simulink model "LT_p2017"  (R2015a)
settings: Solver=ode5  StartTime=0  StopTime=sim_time-1/sr  FixedStep=1/sr  RelTol=1e-3
values from neighbouring files (symbols this model uses):
  par = p.Results.par_fix    [balance_sim.m]
settings Model: Creator=lorenz  LastModifiedBy=lorenz
settings DataIOCC: LimitDataPoints=off  SignalLoggingSaveFormat=ModelDataLogs  SaveOutput=off  SignalLogging=off  DSMLogging=off  SaveTime=off
settings OptimizationCC: OptimizeBlockIOStorage=off  BufferReuse=off  GlobalBufferReuse=off  ExpressionFolding=off  LocalBlockOutputs=off
settings DebuggingCC: UnderspecifiedInitializationDetection=Classic  SolverPrmCheckMsg=warning  InheritedTsInSrcMsg=none  MultiTaskDSMMsg=warning  MultiTaskCondExecSysMsg=none
settings ModelReferenceCC: UpdateModelReferenceTargets=AssumeUpToDate  CheckModelReferenceTargetMessage=warning
settings RTWCC: ProfileTLC=on  RTWUseSimCustomCode=on
settings CodeAppCC: MATLABSourceComments=on

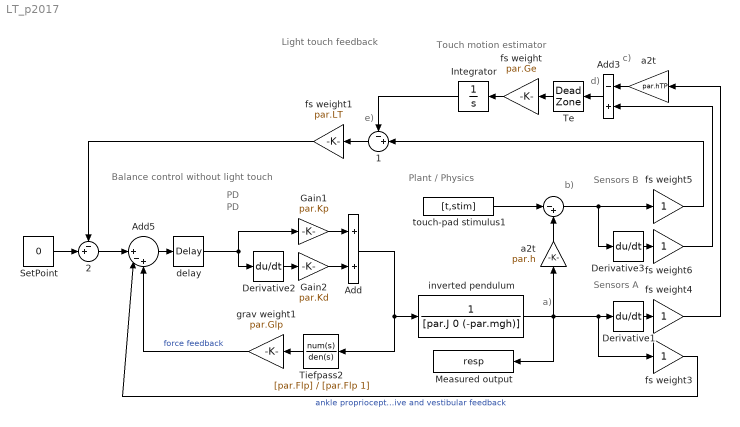
== system LT_p2017 ==
  note: d)
  note: e)
  note: c)
  note: b)
  note: a)
  note: PD
  note: Plant / Physics
  note: Sensors A
  note: Sensors B
  note: Balance control without light touch
  note: PD
  note: Light touch feedback
  note: Touch motion estimator
  " " : Sum  Inputs=|-+
  " 1" : Sum  Inputs=-+|
  " 2" : Sum  Inputs=-+|
  Add : Sum
  Add3 : Sum  Inputs=-+
  Add5 : Sum  Inputs=||+-+
  Derivative1 : Derivative
  Derivative2 : Derivative
  Derivative3 : Derivative
  Gain1 : Gain  Gain=par.Kp
  Gain2 : Gain  Gain=par.Kd
  Integrator : Integrator
  Measured output : ToWorkspace  VariableName=resp  SampleTime=-1
      mask Display: fprintf('measured output')
  SetPoint : Constant  Value=0
  Te : DeadZone  LowerValue=-par.te  UpperValue=par.te  LinearizeAsGain=off
  Tiefpass2 : TransferFcn  Numerator=[par.Flp]  Denominator=[par.Flp 1]
  a2t : Gain  Gain=par.hTP
  "a2t " : Gain  Gain=par.h
  delay : TransportDelay  DelayTime=par.dt  FixedBuffer=on
  fs weight : Gain  Gain=par.Ge
  fs weight1 : Gain  RequirementInfo={} %GIDa_a8373005_bec9_415a_9592_38fc9e9d8428  Gain=par.LT
  fs weight3 : Gain  RequirementInfo={} %GIDa_943181e0_e16f_44fc_af8a_71a118e18fcc
  fs weight4 : Gain  RequirementInfo={} %GIDa_6d4ad6ca_69c9_4f73_8af2_e83a7744f4d6
  fs weight5 : Gain  RequirementInfo={} %GIDa_743b38ee_7318_4b9b_b0be_99d5a1396f7a
  fs weight6 : Gain  RequirementInfo={} %GIDa_91e8bb4a_b572_4304_8634_bbdbe6fba930
  grav weight1 : Gain  Gain=par.Glp
  inverted pendulum : TransferFcn  Denominator=[par.J 0 (-par.mgh)]
  touch-pad stimulus1 : FromWorkspace  VariableName=[t,stim]
      mask Display: fprintf('Stimulus')
  wires:
  Add3/1 -> Te/1
  Derivative1/1 -> fs weight4/1
  Tiefpass2/1 -> grav weight1/1
  SetPoint/1 -> " 2"/2
  Add/1 -> Tiefpass2/1, inverted pendulum/1
  touch-pad stimulus1/1 -> " "/1
  Gain1/1 -> Add/1
  delay/1 -> Gain1/1, Derivative2/1
  Derivative2/1 -> Gain2/1
  Gain2/1 -> Add/2
  grav weight1/1 -> Add5/3  "force feedback"
  Integrator/1 -> " 1"/1
  fs weight1/1 -> " 2"/1
  fs weight3/1 -> Add5/2  "ankle proprioceptive and vestibular feedback"
  fs weight/1 -> Integrator/1
  Te/1 -> fs weight/1
  " 1"/1 -> fs weight1/1
  Add5/1 -> delay/1
  a2t/1 -> Add3/1
  "a2t "/1 -> " "/2
  fs weight4/1 -> a2t/1
  Derivative3/1 -> fs weight6/1
  " "/1 -> Derivative3/1, fs weight5/1
  fs weight6/1 -> Add3/2
  fs weight5/1 -> " 1"/2
  " 2"/1 -> Add5/1
  inverted pendulum/1 -> Measured output/1, fs weight3/1, Derivative1/1, "a2t "/1
